simulink model "da_simulink"  (R2018a)
settings: Solver=ode45  StartTime=0.0  StopTime=2  RelTol=1e-3  EnableMultiTasking=on
values from neighbouring files (symbols this model uses):
  A = [0 1 0 0;20.6 0 0 0;0 0 0 1;-0.5 0 0 0]    [a_ssae.m]
  B = [0;-1;0;0.5]    [a_ssae.m]    (also in e_ssae.m)
  C = [1 0 0 0;0 0 1 0]    [a_ssae.m]    (also in e_ssae.m)
  initial = [-0.2;-0.06;0.01;0.3]    [a_ssae.m]
  K1 = -1*K    [a_ssae.m]
  K4 = [6 0;0 -1392.3;-0.136 0;0 33.6]    [d_ssae.m]
settings Model: Creator=Γιώργος  LastModifiedBy=chron
settings DataIOCC: FinalStateName=xFinald  LimitDataPoints=on  SaveFinalState=on  SaveFormat=Array  SaveState=on  StateSaveName=xoutd  TimeSaveName=toutd  OutputSaveName=youd
settings OptimizationCC: LifeSpan=inf
settings DebuggingCC: SFUnexpectedBacktrackingDiag=warning  SFNoUnconditionalDefaultTransitionDiag=warning  SFExecutionAtInitializationDiag=none
settings HardwareCC: ProdBitPerPointer=32  ProdBitPerSizeT=32  ProdBitPerPtrDiffT=32  ProdLargestAtomicFloat=None  ProdIntDivRoundTo=Undefined  ProdEndianess=Unspecified  ProdWordSize=32  ProdHWDeviceType=32-bit Generic
settings ModelReferenceCC: PropagateSignalLabelsOutOfModel=off
settings CodeAppCC: StateflowObjectComments=on
settings GRTTargetCC: TargetLangStandard=C89/C90 (ANSI)  GeneratePreprocessorConditionals=Disable all
settings ConfigComp: CovMetricSettings=dw  CovHtmlReporting=on  CovSaveCumulativeToWorkspaceVar=on  CovSaveSingleToWorkspaceVar=on  CovExternalEMLEnable=off

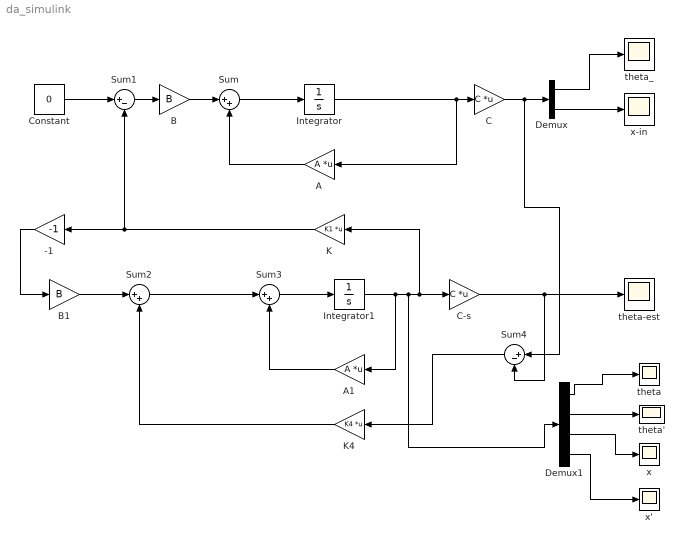
== system da_simulink ==
  -1 : Gain  Gain=-1
  A : Gain  Gain=A  Multiplication=Matrix(K*u)
  A1 : Gain  Gain=A  Multiplication=Matrix(K*u)
  B : Gain  Gain=B
  B1 : Gain  Gain=B
  C : Gain  Gain=C  Multiplication=Matrix(K*u) (u vector)
  C-s : Gain  Gain=C  Multiplication=Matrix(K*u) (u vector)
  Constant : Constant  Value=0
  Demux : Demux  Outputs=2
  Demux1 : Demux
  Integrator : Integrator  InitialCondition=initial
  Integrator1 : Integrator  InitialCondition=initial
  K : Gain  Gain=K1  Multiplication=Matrix(K*u)
  K4 : Gain  Gain=K4  Multiplication=Matrix(K*u)
  Sum : Sum  Inputs=|++
  Sum1 : Sum  Inputs=|+-
  Sum2 : Sum  Inputs=|++
  Sum3 : Sum  Inputs=|++
  Sum4 : Sum  Inputs=|+-
  theta : Scope
  theta' : Scope
  theta-est : Scope
  theta_ : Scope
  x : Scope
  "x' " : Scope
  x-in : Scope
  wires:
  C/1 -> Sum4/1, Demux/1
  Demux/1 -> theta_/1
  A/1 -> Sum/2
  Sum/1 -> Integrator/1
  Sum1/1 -> B/1
  B/1 -> Sum/1
  Integrator/1 -> A/1, C/1
  K/1 -> -1/1, Sum1/2
  Sum3/1 -> Integrator1/1
  Integrator1/1 -> A1/1, Demux1/1, K/1, C-s/1
  C-s/1 -> theta-est/1, Sum4/2
  K4/1 -> Sum2/2
  A1/1 -> Sum3/2
  Demux/2 -> x-in/1
  Sum4/1 -> K4/1
  Sum2/1 -> Sum3/1
  Constant/1 -> Sum1/1
  B1/1 -> Sum2/1
  -1/1 -> B1/1
  Demux1/1 -> theta/1
  Demux1/2 -> theta'/1
  Demux1/3 -> x/1
  Demux1/4 -> "x' "/1
